simulink model "controller_model"  (R2016a)
settings: Solver=ode4  SolverMode=SingleTasking  StartTime=0.0  StopTime=tend  FixedStep=dt_rths  RelTol=1e-3
values from neighbouring files (symbols this model uses):
  dt_rths = 1/fs    (= 0.000244140625)    [A1_main_SMC.m]    (also in A2_main_PI.m; A4_Plots.m)
  sat_limit_lower = -3.8    [F1_input_file.m]
  sat_limit_upper = +3.8    (= 3.8)    [F1_input_file.m]
undefined symbols (not defined in the file or in its folder): Acd, Apred, Bcd, Bpred, Ccd, Cpred, Dcd, Dpred
settings Model: Creator=Sandra  LastModifiedBy=user
settings DataIOCC: SaveFormat=StructureWithTime
settings DebuggingCC: InheritedTsInSrcMsg=none  SFUnexpectedBacktrackingDiag=error  SFNoUnconditionalDefaultTransitionDiag=error
settings HardwareCC: ProdWordSize=32  ProdHWDeviceType=Specified
settings ModelReferenceCC: EnableRefExpFcnMdlSchedulingChecks=off
settings GRTTargetCC: TargetLangStandard=C99 (ISO)
settings ConfigComp: CovMetricSettings=dwe  CovSaveCumulativeToWorkspaceVar=off  CovSaveSingleToWorkspaceVar=off  CovExternalEMLEnable=on

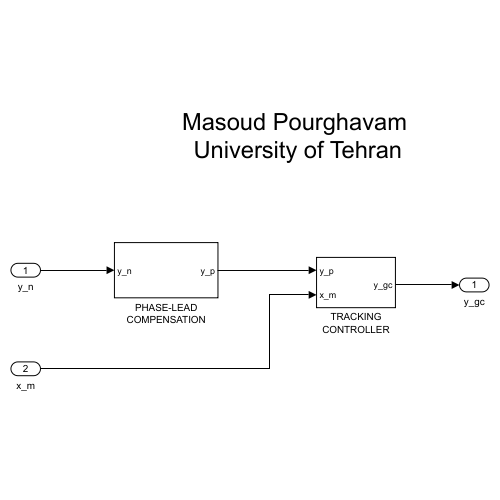
[thumbnail: Simulink's stored preview of the top-level diagram]
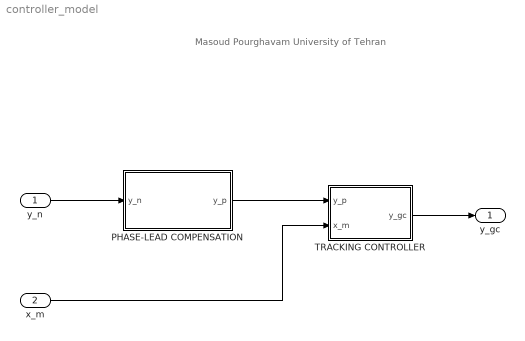
== system controller_model ==
  note: Masoud Pourghavam
      | University of Tehran
  y_n : Inport
  x_m : Inport  Port=2
  PHASE-LEAD COMPENSATION : Subsystem
  TRACKING CONTROLLER : Subsystem
  y_gc : Outport
  wires:
  TRACKING CONTROLLER/1(y_gc) -> y_gc/1
  PHASE-LEAD COMPENSATION/1(y_p) -> TRACKING CONTROLLER/1(y_p)
  y_n/1 -> PHASE-LEAD COMPENSATION/1(y_n)
  x_m/1 -> TRACKING CONTROLLER/2(x_m)

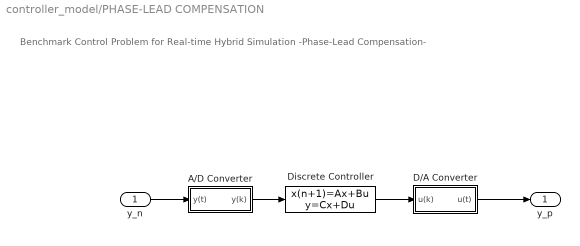
== system controller_model/PHASE-LEAD COMPENSATION ==
  note: Benchmark Control Problem for Real-time Hybrid Simulation
      | -Phase-Lead Compensation-
  y_n : Inport
  A/D Converter : Subsystem
  D/A Converter : Subsystem
  Discrete Controller : DiscreteStateSpace  A=Apred  B=Bpred  C=Cpred  D=Dpred  SampleTime=dt_rths
  y_p : Outport
  wires:
  Discrete Controller/1 -> D/A Converter/1(u(k))
  y_n/1 -> A/D Converter/1(y(t))
  A/D Converter/1(y(k)) -> Discrete Controller/1
  D/A Converter/1(u(t)) -> y_p/1

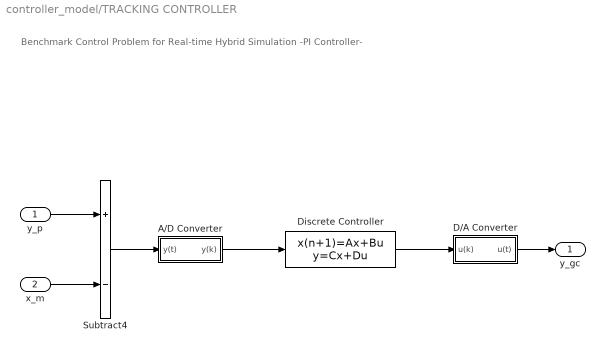
== system controller_model/TRACKING CONTROLLER ==
  note: Benchmark Control Problem for Real-time Hybrid Simulation
      | -PI Controller-
  y_p : Inport
  x_m : Inport  Port=2
  A/D Converter : Subsystem
  D/A Converter : Subsystem
  Discrete Controller : DiscreteStateSpace  A=Acd  B=Bcd  C=Ccd  D=Dcd  SampleTime=dt_rths
  Subtract4 : Sum  Inputs=+-
  y_gc : Outport
  wires:
  y_p/1 -> Subtract4/1
  Discrete Controller/1 -> D/A Converter/1(u(k))
  Subtract4/1 -> A/D Converter/1(y(t))
  x_m/1 -> Subtract4/2
  A/D Converter/1(y(k)) -> Discrete Controller/1
  D/A Converter/1(u(t)) -> y_gc/1

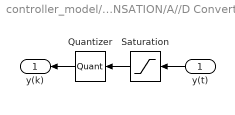
== system controller_model/PHASE-LEAD COMPENSATION/A//D Converter ==
  y(t) : Inport
  Quantizer : Quantizer  QuantizationInterval=quantize_int
  Saturation : Saturate  UpperLimit=sat_limit_upper  LowerLimit=sat_limit_lower
  y(k) : Outport
  wires:
  Saturation/1 -> Quantizer/1
  Quantizer/1 -> y(k)/1
  y(t)/1 -> Saturation/1

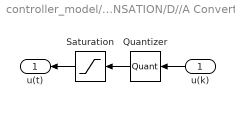
== system controller_model/PHASE-LEAD COMPENSATION/D//A Converter ==
  u(k) : Inport
  Quantizer : Quantizer  QuantizationInterval=quantize_int
  Saturation : Saturate  UpperLimit=sat_limit_upper  LowerLimit=sat_limit_lower
  u(t) : Outport
  wires:
  Saturation/1 -> u(t)/1
  Quantizer/1 -> Saturation/1
  u(k)/1 -> Quantizer/1

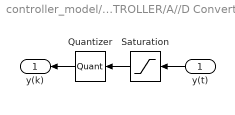
== system controller_model/TRACKING CONTROLLER/A//D Converter ==
  y(t) : Inport
  Quantizer : Quantizer  QuantizationInterval=quantize_int
  Saturation : Saturate  UpperLimit=sat_limit_upper  LowerLimit=sat_limit_lower
  y(k) : Outport
  wires:
  Saturation/1 -> Quantizer/1
  Quantizer/1 -> y(k)/1
  y(t)/1 -> Saturation/1

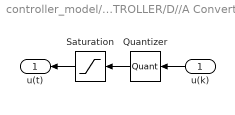
== system controller_model/TRACKING CONTROLLER/D//A Converter ==
  u(k) : Inport
  Quantizer : Quantizer  QuantizationInterval=quantize_int
  Saturation : Saturate  UpperLimit=sat_limit_upper  LowerLimit=sat_limit_lower
  u(t) : Outport
  wires:
  Saturation/1 -> u(t)/1
  Quantizer/1 -> Saturation/1
  u(k)/1 -> Quantizer/1
